simulink model "Quadcopter_BLDC_Mixer"  (R2024a)
settings: Solver=ode45  StartTime=0.0  StopTime=10  RelTol=1e-3
libraries: simulink x1
settings Model: Creator=Pranav Lakshmanan  LastModifiedBy=Pranav Lakshmanan

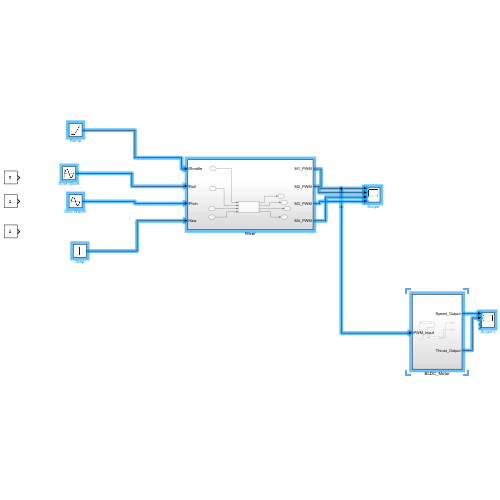
[thumbnail: Simulink's stored preview of the top-level diagram]
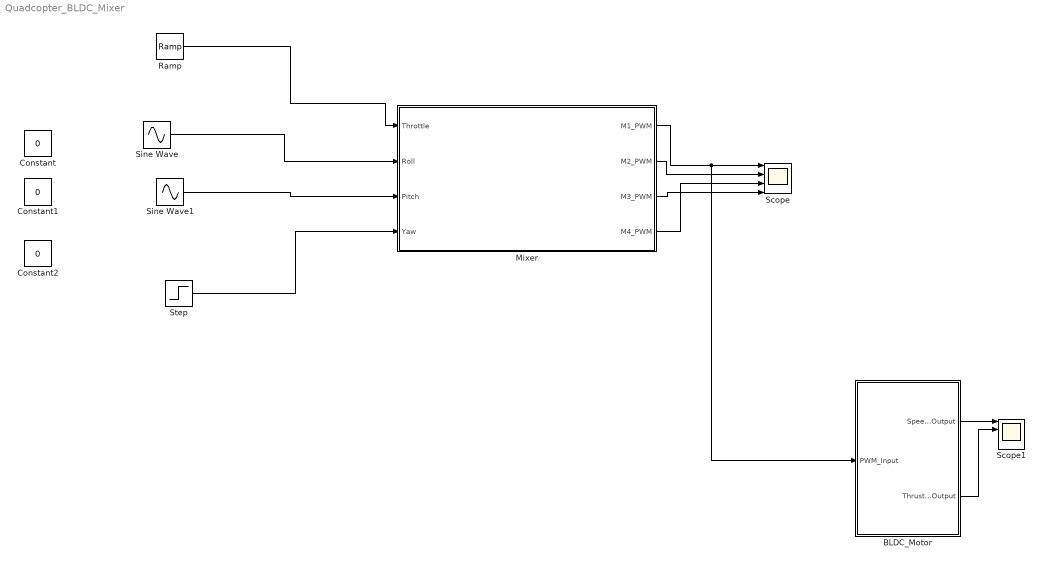
== system Quadcopter_BLDC_Mixer ==
  BLDC_Motor : Subsystem
  Constant : Constant  Value=0
  Constant1 : Constant  Value=0
  Constant2 : Constant  Value=0
  Mixer : Subsystem
  Ramp : simulink/Sources/Ramp  slope=0.2  start=1  InitialOutput=0
  Scope : Scope  NumInputPorts=4
  Scope1 : Scope  NumInputPorts=4
  Sine Wave : Sin  Amplitude=0.3  SampleTime=0
  Sine Wave1 : Sin  Amplitude=0.3  Frequency=0.5  Phase=90  SampleTime=0
  Step : Step  Time=3  After=0.2  SampleTime=0
  wires:
  Mixer/1(M1_PWM) -> BLDC_Motor/1(PWM_Input), Scope/1
  Mixer/2(M2_PWM) -> Scope/2
  Mixer/3(M3_PWM) -> Scope/4
  Mixer/4(M4_PWM) -> Scope/3
  Ramp/1 -> Mixer/1(Throttle)
  Sine Wave/1 -> Mixer/2(Roll)
  Sine Wave1/1 -> Mixer/3(Pitch)
  Step/1 -> Mixer/4(Yaw)
  BLDC_Motor/1(Speed_Output) -> Scope1/1
  BLDC_Motor/2(Thrust_Output) -> Scope1/2

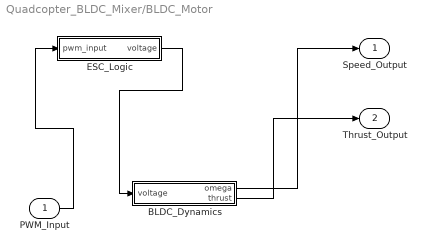
== system Quadcopter_BLDC_Mixer/BLDC_Motor ==
  PWM_Input : Inport
  BLDC_Dynamics : MATLAB Function  TreatAsAtomicUnit=on
  ESC_Logic : MATLAB Function  TreatAsAtomicUnit=on
  Speed_Output : Outport
  Thrust_Output : Outport  Port=2
  wires:
  PWM_Input/1 -> ESC_Logic/1(pwm_input)
  ESC_Logic/1(voltage) -> BLDC_Dynamics/1(voltage)
  BLDC_Dynamics/1(omega) -> Speed_Output/1
  BLDC_Dynamics/2(thrust) -> Thrust_Output/1

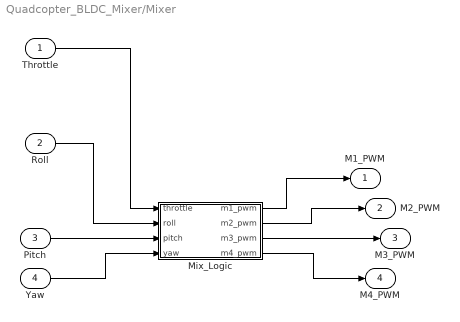
== system Quadcopter_BLDC_Mixer/Mixer ==
  Throttle : Inport
  Roll : Inport  Port=2
  Pitch : Inport  Port=3
  Yaw : Inport  Port=4
  Mix_Logic : MATLAB Function  TreatAsAtomicUnit=on
  M1_PWM : Outport
  M2_PWM : Outport  Port=2
  M3_PWM : Outport  Port=3
  M4_PWM : Outport  Port=4
  wires:
  Throttle/1 -> Mix_Logic/1(throttle)
  Yaw/1 -> Mix_Logic/4(yaw)
  Pitch/1 -> Mix_Logic/3(pitch)
  Roll/1 -> Mix_Logic/2(roll)
  Mix_Logic/4(m4_pwm) -> M4_PWM/1
  Mix_Logic/3(m3_pwm) -> M3_PWM/1
  Mix_Logic/2(m2_pwm) -> M2_PWM/1
  Mix_Logic/1(m1_pwm) -> M1_PWM/1

== matlab function Quadcopter_BLDC_Mixer/BLDC_Motor/BLDC_Dynamics ==
  data: voltage input; omega output; thrust output
function [omega, thrust] = fcn(voltage)
    persistent curr_omega i_q;
    if isempty(curr_omega)
        curr_omega = 0;
        i_q = 0;
    end
    
    % Motor parameters
    Rs = 0.135;      % Stator resistance (Ohm)
    Ls = 0.000169;   % Stator inductance (H)
    Ke = 0.0136;     % Back-EMF constant (V/rad/s)
    Kt = 0.0136;     % Torque constant (N-m/A)
    J = 0.0000135;   % Rotor inertia (kg-m^2)
    B = 0.000000916; % Viscous friction (N-m-s/rad)
    
    Ts = 0.001; % 1kHz simulation rate
    
    % Back-EMF
    bemf = Ke * curr_omega;
    
    % Q-axis current dynamics
    di_q = (voltage - Rs*i_q - bemf)/Ls;
    i_q = i_q + di_q*Ts;
    
    % Torque calculation
    Te = Kt * i_q;
    
    % Mechanical dynamics
    domega = (Te - B*curr_omega)/J;
    curr_omega = curr_omega + domega*Ts;
    
    % Calculate thrust
    Kt_prop = 1.1e-6; % Propeller thrust coefficient
    thrust = Kt_prop * curr_omega^2;
    
    % Outputs
    omega = curr_omega;
end

== matlab function Quadcopter_BLDC_Mixer/BLDC_Motor/ESC_Logic ==
  data: pwm_input input; voltage output
function voltage = fcn(pwm_input)
    % Convert PWM (1000-2000us) to voltage (0-12V)
    min_pwm = 1000;
    max_pwm = 2000;
    max_voltage = 12;
    
    % Normalize PWM input
    duty_cycle = (pwm_input - min_pwm)/(max_pwm - min_pwm);
    duty_cycle = max(0, min(1, duty_cycle));
    
    % Convert to voltage
    voltage = duty_cycle * max_voltage;
end

== matlab function Quadcopter_BLDC_Mixer/Mixer/Mix_Logic ==
  data: throttle input; m1_pwm output; roll input; pitch input; yaw input; m2_pwm output; m3_pwm output; m4_pwm output
function [m1_pwm, m2_pwm, m3_pwm, m4_pwm] = fcn(throttle, roll, pitch, yaw)
    % Convert normalized inputs (-1 to 1) to PWM (1000-2000)
    base_pwm = 1000;
    pwm_range = 1000;
    
    % Mixing matrix
    % Motor arrangement:
    %   M2   M1
    %     \ /
    %     / \
    %   M3   M4
    
    m1_pwm = base_pwm + pwm_range * (throttle + roll + pitch - yaw);  % Front Right
    m2_pwm = base_pwm + pwm_range * (throttle - roll + pitch + yaw);  % Front Left
    m3_pwm = base_pwm + pwm_range * (throttle - roll - pitch - yaw);  % Rear Left
    m4_pwm = base_pwm + pwm_range * (throttle + roll - pitch + yaw);  % Rear Right
    
    % Constrain outputs
    m1_pwm = max(1000, min(2000, m1_pwm));
    m2_pwm = max(1000, min(2000, m2_pwm));
    m3_pwm = max(1000, min(2000, m3_pwm));
    m4_pwm = max(1000, min(2000, m4_pwm));
end
